simulink model "nms_model"  (R2020a)
settings: Solver=ode15s  StartTime=0.0  StopTime=2.6  MaxStep=.01  RelTol=1e-4  AbsTol=1e-6  EnableMultiTasking=on
values from neighbouring files (symbols this model uses):
  dt_visual = -1    [NMScontrol.m]    (also in runmodel.m = 0.001)
  g = params.g    [NMPCcostFunction.m]    (also in dynamicsNMPC.m = 9.81)
  m = parametersOpt(1)    [CGBgreybox.m]    (also in NMPCcostFunction.m = params.m)
undefined symbols (not defined in the file or in its folder): hatLeftHipToCenterDistWidth, initialTargetAngle, LongDelay, LongLoopDelay, LPreStimBFSHinit, LPreStimGASinit, LPreStimGLUinit, LPreStimHABinit, LPreStimHADinit, LPreStimHAMinit, LPreStimHFLinit, LPreStimRFinit, LPreStimSOLinit, LPreStimTAinit, LPreStimVASinit, LTargetAngleInit, LTargetAngleRInit, MidDelay, RPreStimBFSHinit, RPreStimGASinit, RPreStimGLUinit, RPreStimHABinit, RPreStimHADinit, RPreStimHAMinit, RPreStimHFLinit, RPreStimRFinit, RPreStimSOLinit, RPreStimTAinit, RPreStimVASinit, RTargetAngleInit, RTargetAngleRInit, ShortDelay, termination_height, thetaHATref, X, Y, Z
libraries: NeuroMuscularLibrary x107, nesl_utility x25, sm_lib x16, simulink x3
(part 1 of 3)
settings Model: SimulationMode=rapid-accelerator  ParamWorkspaceSource=ReferencedWorkspace  ExtModeTrigDuration=100  TunableVars=GainGAS,GainGLU,GainHAM,GainKneeOverExt,GainSOL,GainSOLTA,GainTA,GainVAS,Kglu,PosGainGG,SpeedGainGG,groundTheta,groundX,groundZ,hipDGain,hipPGain,kneeExtendGain,kneeFlexGain,kneeHoldGain1,kneeHoldGain2,kneeStopGain,legAngleFilter,legLengthClr,simbiconGainD,simbiconGainV,simbiconLegAngle0  TunableVarsStorageClass=Auto,Auto,Auto,Auto,Auto,Auto,Auto,Auto,Auto,Auto,Auto,Auto,Auto,Auto,Auto,Auto,Auto,Auto,Auto,Auto,Auto,Auto,Auto,Auto,Auto,Auto  TunableVarsTypeQualifier=,,,,,,,,,,,,,,,,,,,,,,,,,  Creator=nitisht  LastModifiedBy=Jesper
settings SolverCC: AutoScaleAbsTol=off  ZeroCrossAlgorithm=Adaptive
settings DataIOCC: LimitDataPoints=on  SaveFinalState=on  SaveFormat=StructureWithTime  SaveOutput=off  SaveState=on  ReturnWorkspaceOutputs=off  StateSaveName=tmp_raccel_xout  SignalLoggingName=tmp_raccel_logsout
settings OptimizationCC: DefaultParameterBehavior=Inlined  EfficientMapNaN2IntZero=off  LifeSpan=inf  SimCompilerOptimization=on
settings DebuggingCC: SaveWithDisabledLinksMsg=none  UnderspecifiedInitializationDetection=Classic  MergeDetectMultiDrivingBlocksExec=none  IgnoredZcDiagnostic=none  SolverPrmCheckMsg=warning  StateNameClashWarn=warning  SFUnexpectedBacktrackingDiag=warning  SFNoUnconditionalDefaultTransitionDiag=warning  SFExecutionAtInitializationDiag=none  ArithmeticOperatorsInVariantConditions=warning
settings HardwareCC: ProdBitPerPointer=32  ProdBitPerSizeT=32  ProdBitPerPtrDiffT=32  ProdLargestAtomicFloat=None  ProdIntDivRoundTo=Undefined  ProdEndianess=Unspecified  ProdWordSize=32  ProdHWDeviceType=Generic->Unspecified (assume 32-bit Generic)  TargetBitPerPointer=64  TargetBitPerSizeT=64  TargetBitPerPtrDiffT=64  TargetLongLongMode=on  TargetIntDivRoundTo=Zero  TargetEndianess=LittleEndian  TargetWordSize=64  TargetHWDeviceType=MATLAB Host  ProdEqTarget=off
settings ModelReferenceCC: PropagateSignalLabelsOutOfModel=off
settings SFSimCC: SFSimEcho=off  SimUseLocalCustomCode=off  CustomCodeUndefinedFunction=UseInterfaceOnly
settings RTWCC: SystemTargetFile=raccel.tlc  TemplateMakefile=raccel_default_tmf  RTWUseLocalCustomCode=off  RTWUseSimCustomCode=on
settings CodeAppCC: GenerateComments=off  MaxIdLength=128  MangleLength=10  SimulinkBlockComments=off
settings RaccelTargetCC: MultiInstanceERTCode=off  ENABLE_SLEXEC_SSBRIDGE=0  RTWCAPIParams=off  RTWCAPIRootIO=off
settings ConfigComp: CovMetricSettings=dw  CovHtmlReporting=on  CovSaveCumulativeToWorkspaceVar=on  CovSaveSingleToWorkspaceVar=on  CovExternalEMLEnable=off  CovSFcnEnable=off
settings SimscapeCC: SimscapeNormalizeSystem=off
settings ConfigurationSet: Description=SimMechanics 2G

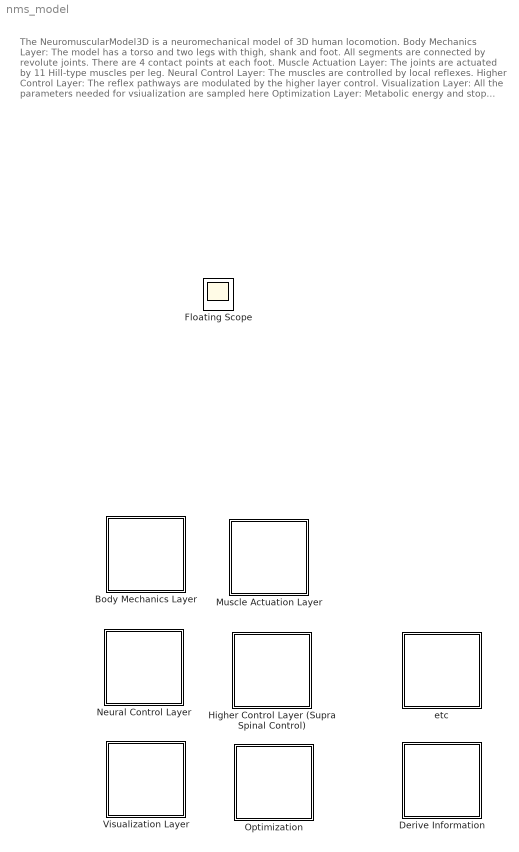
== system nms_model ==
  note: The NeuromuscularModel3D is a neuromechanical model of 3D human locomotion.
      |
      | Body Mechanics Layer:
      | The model has a torso and two legs with thigh, shank and foot.
      | All segments are connected by revolute joints.
      | There are 4 contact points at each foot.
      |
      | Muscle Actuation Layer:
      | The joints are actuated by 11 Hill-type muscles per leg.
      |
      | Neural Control Layer:
      | The muscles are controlled by local reflexes.
      |
      | Higher Control Layer:
      | The reflex pathways are modulated by the higher layer control.
      |
      | Visualization Layer:
      | All the parameters needed for vsiualization are sampled here
      |
      | Optimization Layer:
      | Metabolic energy and stop torques are calculated here.
      |
      | Derive Information Layer:
      | Contains gait phase detector, self collision detector, and step information calculator.
      |
      | Etc Layer:
      | Contains some stop conditions for when to stop simulation.
  Body Mechanics Layer : Subsystem
  Derive Information : Subsystem
  Higher Control Layer (Supra Spinal Control) : Subsystem
  Muscle Actuation Layer : Subsystem
  Neural Control Layer : Subsystem
  Optimization : Subsystem
  Visualization Layer : Subsystem
  etc : Subsystem
  Floating Scope : Scope

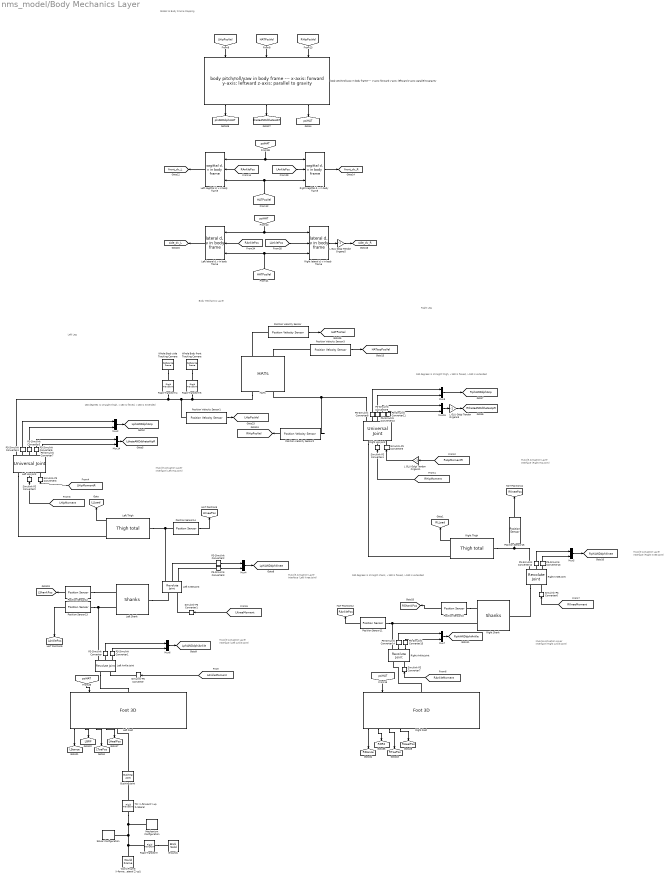
== system nms_model/Body Mechanics Layer ==
  note: 180 degrees is straight thigh, <180 is flexed, >180 is extended
  note: Body Mechanics Layer
  note: Left Leg
  note: Right Leg
  note: Muscle Actuation
      | Layer Interface
      | (Left Hip Joint)
  note: Muscle Actuation
      | Layer Interface
      | (Left Knee Joint)
  note: Muscle Actuation
      | Layer Interface
      | (Left Ankle Joint)
  note: Muscle Actuation
      | Layer Interface
      | (Right Ankle Joint)
  note: Muscle Actuation
      | Layer Interface
      | (Right Knee Joint)
  note: Muscle Actuation
      | Layer Interface
      | (Right Hip Joint)
  note: Global to Body Frame Mapping
  note: 180 degrees is straight thigh, <180 is flexed, >180 is extended
  note: 180 degrees is straight shank, <180 is flexed, >180 is extended
  Bushing Joint : sm_lib/Joints/Bushing Joint  JointMode=Normal  SenseConstraintForce=off  SenseConstraintForceX=off  SenseConstraintForceY=off  SenseConstraintForceZ=off  SenseConstraintTorque=off  SenseConstraintTorqueX=off  SenseConstraintTorqueY=off  SenseConstraintTorqueZ=off  SenseTotalForce=off  SenseTotalForceX=off  SenseTotalForceY=off  SenseTotalForceZ=off  SenseTotalTorque=off  SenseTotalTorqueX=off  SenseTotalTorqueY=off  SenseTotalTorqueZ=off  CompositeWrenchDir=FollowerOnBase  CompositeWrenchFrame=BaseFrame  PxEquilibriumPosition=0  PxEquilibriumPositionUnits=m  PxSpringStiffness=0  PxSpringStiffnessUnits=N/m  PxDampingCoefficient=0  PxDampingCoefficientUnits=N/(m/s)  PxTorqueActuationMode=NoTorque  PxMotionActuationMode=ComputedMotion  PxSensePosition=off  PxSenseVelocity=off  PxSenseAcceleration=off  PxSenseTorqueForce=off  PxSenseLowerLimitTorqueForce=off  PxSenseUpperLimitTorqueForce=off  PxLowerLimitSpecify=off  PxLowerLimitBound=-1  PxLowerLimitBoundUnits=m  PxLowerLimitStiffness=1e6  PxLowerLimitStiffnessUnits=N/m  PxLowerLimitDamping=1e3  PxLowerLimitDampingUnits=N/(m/s)  PxLowerLimitTransitionRegionWidth=1e-4  PxLowerLimitTransitionRegionWidthUnits=m  PxUpperLimitSpecify=off  PxUpperLimitBound=1  PxUpperLimitBoundUnits=m  PxUpperLimitStiffness=1e6  PxUpperLimitStiffnessUnits=N/m  PxUpperLimitDamping=1e3  PxUpperLimitDampingUnits=N/(m/s)  PxUpperLimitTransitionRegionWidth=1e-4  PxUpperLimitTransitionRegionWidthUnits=m  PxPositionTargetSpecify=on  PxPositionTargetPriority=High  PxPositionTargetValue=xInit  PxPositionTargetValueUnits=m  PxVelocityTargetSpecify=on  PxVelocityTargetPriority=High  PxVelocityTargetValue=vxInit  PxVelocityTargetValueUnits=m/s  PyEquilibriumPosition=0  PyEquilibriumPositionUnits=m  PySpringStiffness=0  PySpringStiffnessUnits=N/m  PyDampingCoefficient=0  PyDampingCoefficientUnits=N/(m/s)  PyTorqueActuationMode=NoTorque  PyMotionActuationMode=ComputedMotion  PySensePosition=off  PySenseVelocity=off  PySenseAcceleration=off  PySenseTorqueForce=off  PySenseLowerLimitTorqueForce=off  PySenseUpperLimitTorqueForce=off  PyLowerLimitSpecify=off  PyLowerLimitBound=-1  PyLowerLimitBoundUnits=m  PyLowerLimitStiffness=1e6  PyLowerLimitStiffnessUnits=N/m  PyLowerLimitDamping=1e3  PyLowerLimitDampingUnits=N/(m/s)  PyLowerLimitTransitionRegionWidth=1e-4  PyLowerLimitTransitionRegionWidthUnits=m  PyUpperLimitSpecify=off  PyUpperLimitBound=1  PyUpperLimitBoundUnits=m  PyUpperLimitStiffness=1e6  PyUpperLimitStiffnessUnits=N/m  PyUpperLimitDamping=1e3  PyUpperLimitDampingUnits=N/(m/s)  PyUpperLimitTransitionRegionWidth=1e-4  PyUpperLimitTransitionRegionWidthUnits=m  PyPositionTargetSpecify=on  PyPositionTargetPriority=High  PyPositionTargetValue=zInit  PyPositionTargetValueUnits=m  PyVelocityTargetSpecify=on  PyVelocityTargetPriority=High  PyVelocityTargetValue=vzInit  PyVelocityTargetValueUnits=m/s  PzEquilibriumPosition=0  PzEquilibriumPositionUnits=m  PzSpringStiffness=0  PzSpringStiffnessUnits=N/m  PzDampingCoefficient=0  PzDampingCoefficientUnits=N/(m/s)  PzTorqueActuationMode=NoTorque  PzMotionActuationMode=ComputedMotion  PzSensePosition=off  PzSenseVelocity=off  PzSenseAcceleration=off  PzSenseTorqueForce=off  PzSenseLowerLimitTorqueForce=off  PzSenseUpperLimitTorqueForce=off  PzLowerLimitSpecify=off  PzLowerLimitBound=-1  PzLowerLimitBoundUnits=m  PzLowerLimitStiffness=1e6  PzLowerLimitStiffnessUnits=N/m  PzLowerLimitDamping=1e3  PzLowerLimitDampingUnits=N/(m/s)  PzLowerLimitTransitionRegionWidth=1e-4  PzLowerLimitTransitionRegionWidthUnits=m  PzUpperLimitSpecify=off  PzUpperLimitBound=1  PzUpperLimitBoundUnits=m  PzUpperLimitStiffness=1e6  PzUpperLimitStiffnessUnits=N/m  PzUpperLimitDamping=1e3  PzUpperLimitDampingUnits=N/(m/s)  PzUpperLimitTransitionRegionWidth=1e-4  PzUpperLimitTransitionRegionWidthUnits=m  PzPositionTargetSpecify=on  PzPositionTargetPriority=High  PzPositionTargetValue=yInit  PzPositionTargetValueUnits=m  PzVelocityTargetSpecify=on  PzVelocityTargetPriority=High  PzVelocityTargetValue=vyInit  PzVelocityTargetValueUnits=m/s  RxEquilibriumPosition=0  RxEquilibriumPositionUnits=deg  RxSpringStiffness=0  RxSpringStiffnessUnits=N*m/deg  RxDampingCoefficient=0  RxDampingCoefficientUnits=N*m/(deg/s)  RxTorqueActuationMode=NoTorque  RxMotionActuationMode=ComputedMotion  RxSensePosition=off  RxSenseVelocity=off  RxSenseAcceleration=off  RxSenseTorqueForce=off  RxSenseLowerLimitTorqueForce=off  RxSenseUpperLimitTorqueForce=off  RxLowerLimitSpecify=off  RxLowerLimitBound=-90  RxLowerLimitBoundUnits=deg  RxLowerLimitStiffness=1e4  RxLowerLimitStiffnessUnits=N*m/deg  RxLowerLimitDamping=10  RxLowerLimitDampingUnits=N*m/(deg/s)  RxLowerLimitTransitionRegionWidth=0.1  RxLowerLimitTransitionRegionWidthUnits=deg  RxUpperLimitSpecify=off  RxUpperLimitBound=90  RxUpperLimitBoundUnits=deg  RxUpperLimitStiffness=1e4  RxUpperLimitStiffnessUnits=N*m/deg  RxUpperLimitDamping=10  RxUpperLimitDampingUnits=N*m/(deg/s)  RxUpperLimitTransitionRegionWidth=0.1  RxUpperLimitTransitionRegionWidthUnits=deg  RxPositionTargetSpecify=on  RxPositionTargetPriority=High  RxPositionTargetValue=rollInit  RxPositionTargetValueUnits=rad  RxVelocityTargetSpecify=on  RxVelocityTargetPriority=High  RxVelocityTargetValue=0  RxVelocityTargetValueUnits=rad/s  RyEquilibriumPosition=0  RyEquilibriumPositionUnits=deg  RySpringStiffness=0  RySpringStiffnessUnits=N*m/deg  RyDampingCoefficient=0  RyDampingCoefficientUnits=N*m/(deg/s)  RyTorqueActuationMode=NoTorque  RyMotionActuationMode=ComputedMotion  RySensePosition=off  RySenseVelocity=off  RySenseAcceleration=off  RySenseTorqueForce=off  RySenseLowerLimitTorqueForce=off  RySenseUpperLimitTorqueForce=off  RyLowerLimitSpecify=off  RyLowerLimitBound=-90  RyLowerLimitBoundUnits=deg  RyLowerLimitStiffness=1e4  RyLowerLimitStiffnessUnits=N*m/deg  RyLowerLimitDamping=10  RyLowerLimitDampingUnits=N*m/(deg/s)  RyLowerLimitTransitionRegionWidth=0.1  RyLowerLimitTransitionRegionWidthUnits=deg  RyUpperLimitSpecify=off  RyUpperLimitBound=90  RyUpperLimitBoundUnits=deg  RyUpperLimitStiffness=1e4  RyUpperLimitStiffnessUnits=N*m/deg  RyUpperLimitDamping=10  RyUpperLimitDampingUnits=N*m/(deg/s)  RyUpperLimitTransitionRegionWidth=0.1  RyUpperLimitTransitionRegionWidthUnits=deg  RyPositionTargetSpecify=on  RyPositionTargetPriority=High  RyPositionTargetValue=yawInit  RyPositionTargetValueUnits=rad  RyVelocityTargetSpecify=on  RyVelocityTargetPriority=High  RyVelocityTargetValue=0  RyVelocityTargetValueUnits=rad/s  RzEquilibriumPosition=0  RzEquilibriumPositionUnits=deg  RzSpringStiffness=0  RzSpringStiffnessUnits=N*m/deg  RzDampingCoefficient=0  RzDampingCoefficientUnits=N*m/(deg/s)  RzTorqueActuationMode=NoTorque  RzMotionActuationMode=ComputedMotion  RzSensePosition=off  RzSenseVelocity=off  RzSenseAcceleration=off  RzSenseTorqueForce=off  RzSenseLowerLimitTorqueForce=off  RzSenseUpperLimitTorqueForce=off  RzLowerLimitSpecify=off  RzLowerLimitBound=-90  RzLowerLimitBoundUnits=deg  RzLowerLimitStiffness=1e4  RzLowerLimitStiffnessUnits=N*m/deg  RzLowerLimitDamping=10  RzLowerLimitDampingUnits=N*m/(deg/s)  RzLowerLimitTransitionRegionWidth=0.1  RzLowerLimitTransitionRegionWidthUnits=deg  RzUpperLimitSpecify=off  RzUpperLimitBound=90  RzUpperLimitBoundUnits=deg  RzUpperLimitStiffness=1e4  RzUpperLimitStiffnessUnits=N*m/deg  RzUpperLimitDamping=10  RzUpperLimitDampingUnits=N*m/(deg/s)  RzUpperLimitTransitionRegionWidth=0.1  RzUpperLimitTransitionRegionWidthUnits=deg  RzPositionTargetSpecify=off  RzPositionTargetPriority=High  RzPositionTargetValue=0  RzPositionTargetValueUnits=deg  RzVelocityTargetSpecify=off  RzVelocityTargetPriority=High  RzVelocityTargetValue=0  RzVelocityTargetValueUnits=deg/s
  Ground1 : sm_lib/Body Elements/Brick Solid  GraphicAmbientColor=[0.15 0.15 0.15 1.0]  BasedOnType=Density  BrickDimensions=[3 1 .01]  BrickDimensionUnits=m  CenterOfMass=[0 0 0]  CenterOfMassUnits=m  GraphicDiffuseColor=[0.4 0.2 0.0]  Density=1000  DensityUnits=kg/(m^3)  DoExposeReferenceFrame=on  GraphicEmissiveColor=[0.0 0.0 0.0 1.0]  ExportEntireGeometry=off  SerializedFrames=<Frames/>  MarkerShape=Sphere  MarkerSize=10  GraphicType=FromGeometry  InertiaType=Custom  Mass=0  MassUnits=kg  MomentsOfInertia=[0 0 0]  MomentsOfInertiaUnits=kg*m^2  GraphicOpacity=1.0  ProductsOfInertia=[0 0 0]  ProductsOfInertiaUnits=kg*m^2  GraphicShininess=75  GraphicSpecularColor=[0.5 0.5 0.5 1.0]  GraphicVisPropType=SimpleVisualProperties
  HATs : NeuroMuscularLibrary/HATs  SystemSampleTime=-1  Latency=0  AutoFrameSizeCalculation=off
  L GLU Golgi Tendon Organs1 : Gain  Gain=-1
  L GLU Golgi Tendon Organs3 : Gain  Gain=-1
  L GLU Golgi Tendon Organs5 : Gain  Gain=-1
  Left Knee Joint : sm_lib/Joints/Revolute Joint  JointMode=Normal  SenseConstraintForce=off  SenseConstraintForceX=off  SenseConstraintForceY=off  SenseConstraintForceZ=off  SenseConstraintTorque=off  SenseConstraintTorqueX=off  SenseConstraintTorqueY=off  SenseConstraintTorqueZ=off  SenseTotalForce=off  SenseTotalForceX=off  SenseTotalForceY=off  SenseTotalForceZ=off  SenseTotalTorque=off  SenseTotalTorqueX=off  SenseTotalTorqueY=off  SenseTotalTorqueZ=off  CompositeWrenchDir=FollowerOnBase  CompositeWrenchFrame=BaseFrame  EquilibriumPosition=0  EquilibriumPositionUnits=deg  SpringStiffness=0  SpringStiffnessUnits=N*m/deg  DampingCoefficient=0  DampingCoefficientUnits=N*m/(deg/s)  TorqueActuationMode=InputTorque  MotionActuationMode=ComputedMotion  SensePosition=on  SenseVelocity=on  SenseAcceleration=off  SenseTorqueForce=off  SenseLowerLimitTorqueForce=off  SenseUpperLimitTorqueForce=off  LowerLimitSpecify=off  LowerLimitBound=-90  LowerLimitBoundUnits=deg  LowerLimitStiffness=1e4  LowerLimitStiffnessUnits=N*m/deg  LowerLimitDamping=10  LowerLimitDampingUnits=N*m/(deg/s)  LowerLimitTransitionRegionWidth=0.1  LowerLimitTransitionRegionWidthUnits=deg  UpperLimitSpecify=off  UpperLimitBound=90  UpperLimitBoundUnits=deg  UpperLimitStiffness=1e4  UpperLimitStiffnessUnits=N*m/deg  UpperLimitDamping=10  UpperLimitDampingUnits=N*m/(deg/s)  UpperLimitTransitionRegionWidth=0.1  UpperLimitTransitionRegionWidthUnits=deg  PositionTargetSpecify=on  PositionTargetPriority=High  PositionTargetValue=LphiKnee0  PositionTargetValueUnits=rad  VelocityTargetSpecify=on  VelocityTargetPriority=High  VelocityTargetValue=0  VelocityTargetValueUnits=rad/s
  Left Ankle joint : sm_lib/Joints/Revolute Joint  JointMode=Normal  SenseConstraintForce=off  SenseConstraintForceX=off  SenseConstraintForceY=off  SenseConstraintForceZ=off  SenseConstraintTorque=off  SenseConstraintTorqueX=off  SenseConstraintTorqueY=off  SenseConstraintTorqueZ=off  SenseTotalForce=off  SenseTotalForceX=off  SenseTotalForceY=off  SenseTotalForceZ=off  SenseTotalTorque=off  SenseTotalTorqueX=off  SenseTotalTorqueY=off  SenseTotalTorqueZ=off  CompositeWrenchDir=FollowerOnBase  CompositeWrenchFrame=BaseFrame  EquilibriumPosition=0  EquilibriumPositionUnits=deg  SpringStiffness=0  SpringStiffnessUnits=N*m/deg  DampingCoefficient=0  DampingCoefficientUnits=N*m/(deg/s)  TorqueActuationMode=InputTorque  MotionActuationMode=ComputedMotion  SensePosition=on  SenseVelocity=on  SenseAcceleration=off  SenseTorqueForce=off  SenseLowerLimitTorqueForce=off  SenseUpperLimitTorqueForce=off  LowerLimitSpecify=off  LowerLimitBound=-90  LowerLimitBoundUnits=deg  LowerLimitStiffness=1e4  LowerLimitStiffnessUnits=N*m/deg  LowerLimitDamping=10  LowerLimitDampingUnits=N*m/(deg/s)  LowerLimitTransitionRegionWidth=0.1  LowerLimitTransitionRegionWidthUnits=deg  UpperLimitSpecify=off  UpperLimitBound=90  UpperLimitBoundUnits=deg  UpperLimitStiffness=1e4  UpperLimitStiffnessUnits=N*m/deg  UpperLimitDamping=10  UpperLimitDampingUnits=N*m/(deg/s)  UpperLimitTransitionRegionWidth=0.1  UpperLimitTransitionRegionWidthUnits=deg  PositionTargetSpecify=on  PositionTargetPriority=High  PositionTargetValue=LphiAnkle0  PositionTargetValueUnits=rad  VelocityTargetSpecify=on  VelocityTargetPriority=High  VelocityTargetValue=0  VelocityTargetValueUnits=rad/s
  Left Foot : NeuroMuscularLibrary/Foot 3D  footMass=footMass  footInertia=footInertia  footSide=Left foot
  Left Hip Joint : sm_lib/Joints/Universal Joint  JointMode=Normal  SenseConstraintForce=off  SenseConstraintForceX=off  SenseConstraintForceY=off  SenseConstraintForceZ=off  SenseConstraintTorque=off  SenseConstraintTorqueX=off  SenseConstraintTorqueY=off  SenseConstraintTorqueZ=off  SenseTotalForce=off  SenseTotalForceX=off  SenseTotalForceY=off  SenseTotalForceZ=off  SenseTotalTorque=off  SenseTotalTorqueX=off  SenseTotalTorqueY=off  SenseTotalTorqueZ=off  CompositeWrenchDir=FollowerOnBase  CompositeWrenchFrame=BaseFrame  RxEquilibriumPosition=0  RxEquilibriumPositionUnits=deg  RxSpringStiffness=0  RxSpringStiffnessUnits=N*m/deg  RxDampingCoefficient=0  RxDampingCoefficientUnits=N*m/(deg/s)  RxTorqueActuationMode=InputTorque  RxMotionActuationMode=ComputedMotion  RxSensePosition=on  RxSenseVelocity=on  RxSenseAcceleration=off  RxSenseTorqueForce=off  RxSenseLowerLimitTorqueForce=off  RxSenseUpperLimitTorqueForce=off  RxLowerLimitSpecify=off  RxLowerLimitBound=-90  RxLowerLimitBoundUnits=deg  RxLowerLimitStiffness=1e4  RxLowerLimitStiffnessUnits=N*m/deg  RxLowerLimitDamping=10  RxLowerLimitDampingUnits=N*m/(deg/s)  RxLowerLimitTransitionRegionWidth=0.1  RxLowerLimitTransitionRegionWidthUnits=deg  RxUpperLimitSpecify=off  RxUpperLimitBound=90  RxUpperLimitBoundUnits=deg  RxUpperLimitStiffness=1e4  RxUpperLimitStiffnessUnits=N*m/deg  RxUpperLimitDamping=10  RxUpperLimitDampingUnits=N*m/(deg/s)  RxUpperLimitTransitionRegionWidth=0.1  RxUpperLimitTransitionRegionWidthUnits=deg  RxPositionTargetSpecify=on  RxPositionTargetPriority=High  RxPositionTargetValue=LphiHip0  RxPositionTargetValueUnits=rad  RxVelocityTargetSpecify=on  RxVelocityTargetPriority=High  RxVelocityTargetValue=0  RxVelocityTargetValueUnits=rad/s  RyEquilibriumPosition=0  RyEquilibriumPositionUnits=deg  RySpringStiffness=0  RySpringStiffnessUnits=N*m/deg  RyDampingCoefficient=0  RyDampingCoefficientUnits=N*m/(deg/s)  RyTorqueActuationMode=InputTorque  RyMotionActuationMode=ComputedMotion  RySensePosition=on  RySenseVelocity=on  RySenseAcceleration=off  RySenseTorqueForce=off  RySenseLowerLimitTorqueForce=off  RySenseUpperLimitTorqueForce=off  RyLowerLimitSpecify=off  RyLowerLimitBound=-90  RyLowerLimitBoundUnits=deg  RyLowerLimitStiffness=1e4  RyLowerLimitStiffnessUnits=N*m/deg  RyLowerLimitDamping=10  RyLowerLimitDampingUnits=N*m/(deg/s)  RyLowerLimitTransitionRegionWidth=0.1  RyLowerLimitTransitionRegionWidthUnits=deg  RyUpperLimitSpecify=off  RyUpperLimitBound=90  RyUpperLimitBoundUnits=deg  RyUpperLimitStiffness=1e4  RyUpperLimitStiffnessUnits=N*m/deg  RyUpperLimitDamping=10  RyUpperLimitDampingUnits=N*m/(deg/s)  RyUpperLimitTransitionRegionWidth=0.1  RyUpperLimitTransitionRegionWidthUnits=deg  RyPositionTargetSpecify=on  RyPositionTargetPriority=High  RyPositionTargetValue=LphiHipR0  RyPositionTargetValueUnits=rad  RyVelocityTargetSpecify=on  RyVelocityTargetPriority=High  RyVelocityTargetValue=0  RyVelocityTargetValueUnits=rad/s
  Left Shank : NeuroMuscularLibrary/Shanks  SystemSampleTime=-1  Latency=0  AutoFrameSizeCalculation=off
  Left Thigh : NeuroMuscularLibrary/Thigh total  SystemSampleTime=-1  Latency=0  AutoFrameSizeCalculation=off
  "Left lateral d, v in body frame" : NeuroMuscularLibrary/lateral d, v in body frame  SystemSampleTime=-1  Latency=0  AutoFrameSizeCalculation=off
  "Left sagittal d, v in body frame" : NeuroMuscularLibrary/sagittal d, v in body frame  SystemSampleTime=-1  Latency=0  AutoFrameSizeCalculation=off
  Mechanism Configuration : sm_lib/Utilities/Mechanism Configuration  UniformGravity=Constant  GravityVector=[0 0 -g]  GravityUnits=m/s^2  LinearizationDelta=0.001
  Mux{2..7,14..15} (8 alike) : Mux  Inputs=2
  PS-Simulink Converter{,2,4,6,8,10,12,14} (8 alike) : nesl_utility/PS-Simulink Converter  PhysicalDomain=network_engine_domain  SubClassName=ps_output  LeftPortType=input  RightPortType=output  PseudoPeriodic=off  Frequencies=[]  Unit=rad  AffineConversion=off
  PS-Simulink Converter{1,3,5,7,9,11,13,15} (8 alike) : nesl_utility/PS-Simulink Converter  PhysicalDomain=network_engine_domain  SubClassName=ps_output  LeftPortType=input  RightPortType=output  PseudoPeriodic=off  Frequencies=[]  Unit=rad/s  AffineConversion=off
  Position Sensor{10..15} (6 alike) : NeuroMuscularLibrary/Position Sensor  SystemSampleTime=-1  Latency=0  AutoFrameSizeCalculation=off
  Position Velocity Sensor{,1..3} (4 alike) : NeuroMuscularLibrary/Position Velocity Sensor  SystemSampleTime=-1  Latency=0  AutoFrameSizeCalculation=off
  Right Ankle Joint : sm_lib/Joints/Revolute Joint  JointMode=Normal  SenseConstraintForce=off  SenseConstraintForceX=off  SenseConstraintForceY=off  SenseConstraintForceZ=off  SenseConstraintTorque=off  SenseConstraintTorqueX=off  SenseConstraintTorqueY=off  SenseConstraintTorqueZ=off  SenseTotalForce=off  SenseTotalForceX=off  SenseTotalForceY=off  SenseTotalForceZ=off  SenseTotalTorque=off  SenseTotalTorqueX=off  SenseTotalTorqueY=off  SenseTotalTorqueZ=off  CompositeWrenchDir=FollowerOnBase  CompositeWrenchFrame=BaseFrame  EquilibriumPosition=0  EquilibriumPositionUnits=deg  SpringStiffness=0  SpringStiffnessUnits=N*m/deg  DampingCoefficient=0  DampingCoefficientUnits=N*m/(deg/s)  TorqueActuationMode=InputTorque  MotionActuationMode=ComputedMotion  SensePosition=on  SenseVelocity=on  SenseAcceleration=off  SenseTorqueForce=off  SenseLowerLimitTorqueForce=off  SenseUpperLimitTorqueForce=off  LowerLimitSpecify=off  LowerLimitBound=-90  LowerLimitBoundUnits=deg  LowerLimitStiffness=1e4  LowerLimitStiffnessUnits=N*m/deg  LowerLimitDamping=10  LowerLimitDampingUnits=N*m/(deg/s)  LowerLimitTransitionRegionWidth=0.1  LowerLimitTransitionRegionWidthUnits=deg  UpperLimitSpecify=off  UpperLimitBound=90  UpperLimitBoundUnits=deg  UpperLimitStiffness=1e4  UpperLimitStiffnessUnits=N*m/deg  UpperLimitDamping=10  UpperLimitDampingUnits=N*m/(deg/s)  UpperLimitTransitionRegionWidth=0.1  UpperLimitTransitionRegionWidthUnits=deg  PositionTargetSpecify=on  PositionTargetPriority=High  PositionTargetValue=RphiAnkle0  PositionTargetValueUnits=rad  VelocityTargetSpecify=on  VelocityTargetPriority=High  VelocityTargetValue=0  VelocityTargetValueUnits=rad/s
  Right Foot : NeuroMuscularLibrary/Foot 3D  footMass=footMass  footInertia=footInertia  footSide=Right foot
  Right Hip joint : sm_lib/Joints/Universal Joint  JointMode=Normal  SenseConstraintForce=off  SenseConstraintForceX=off  SenseConstraintForceY=off  SenseConstraintForceZ=off  SenseConstraintTorque=off  SenseConstraintTorqueX=off  SenseConstraintTorqueY=off  SenseConstraintTorqueZ=off  SenseTotalForce=off  SenseTotalForceX=off  SenseTotalForceY=off  SenseTotalForceZ=off  SenseTotalTorque=off  SenseTotalTorqueX=off  SenseTotalTorqueY=off  SenseTotalTorqueZ=off  CompositeWrenchDir=FollowerOnBase  CompositeWrenchFrame=BaseFrame  RxEquilibriumPosition=0  RxEquilibriumPositionUnits=deg  RxSpringStiffness=0  RxSpringStiffnessUnits=N*m/deg  RxDampingCoefficient=0  RxDampingCoefficientUnits=N*m/(deg/s)  RxTorqueActuationMode=InputTorque  RxMotionActuationMode=ComputedMotion  RxSensePosition=on  RxSenseVelocity=on  RxSenseAcceleration=off  RxSenseTorqueForce=off  RxSenseLowerLimitTorqueForce=off  RxSenseUpperLimitTorqueForce=off  RxLowerLimitSpecify=off  RxLowerLimitBound=-90  RxLowerLimitBoundUnits=deg  RxLowerLimitStiffness=1e4  RxLowerLimitStiffnessUnits=N*m/deg  RxLowerLimitDamping=10  RxLowerLimitDampingUnits=N*m/(deg/s)  RxLowerLimitTransitionRegionWidth=0.1  RxLowerLimitTransitionRegionWidthUnits=deg  RxUpperLimitSpecify=off  RxUpperLimitBound=90  RxUpperLimitBoundUnits=deg  RxUpperLimitStiffness=1e4  RxUpperLimitStiffnessUnits=N*m/deg  RxUpperLimitDamping=10  RxUpperLimitDampingUnits=N*m/(deg/s)  RxUpperLimitTransitionRegionWidth=0.1  RxUpperLimitTransitionRegionWidthUnits=deg  RxPositionTargetSpecify=on  RxPositionTargetPriority=High  RxPositionTargetValue=RphiHip0  RxPositionTargetValueUnits=rad  RxVelocityTargetSpecify=on  RxVelocityTargetPriority=High  RxVelocityTargetValue=0  RxVelocityTargetValueUnits=rad/s  RyEquilibriumPosition=0  RyEquilibriumPositionUnits=deg  RySpringStiffness=0  RySpringStiffnessUnits=N*m/deg  RyDampingCoefficient=0  RyDampingCoefficientUnits=N*m/(deg/s)  RyTorqueActuationMode=InputTorque  RyMotionActuationMode=ComputedMotion  RySensePosition=on  RySenseVelocity=on  RySenseAcceleration=off  RySenseTorqueForce=off  RySenseLowerLimitTorqueForce=off  RySenseUpperLimitTorqueForce=off  RyLowerLimitSpecify=off  RyLowerLimitBound=-90  RyLowerLimitBoundUnits=deg  RyLowerLimitStiffness=1e4  RyLowerLimitStiffnessUnits=N*m/deg  RyLowerLimitDamping=10  RyLowerLimitDampingUnits=N*m/(deg/s)  RyLowerLimitTransitionRegionWidth=0.1  RyLowerLimitTransitionRegionWidthUnits=deg  RyUpperLimitSpecify=off  RyUpperLimitBound=90  RyUpperLimitBoundUnits=deg  RyUpperLimitStiffness=1e4  RyUpperLimitStiffnessUnits=N*m/deg  RyUpperLimitDamping=10  RyUpperLimitDampingUnits=N*m/(deg/s)  RyUpperLimitTransitionRegionWidth=0.1  RyUpperLimitTransitionRegionWidthUnits=deg  RyPositionTargetSpecify=on  RyPositionTargetPriority=High  RyPositionTargetValue=RphiHipR0  RyPositionTargetValueUnits=rad  RyVelocityTargetSpecify=on  RyVelocityTargetPriority=High  RyVelocityTargetValue=0  RyVelocityTargetValueUnits=rad/s
  Right Knee joint : sm_lib/Joints/Revolute Joint  JointMode=Normal  SenseConstraintForce=off  SenseConstraintForceX=off  SenseConstraintForceY=off  SenseConstraintForceZ=off  SenseConstraintTorque=off  SenseConstraintTorqueX=off  SenseConstraintTorqueY=off  SenseConstraintTorqueZ=off  SenseTotalForce=off  SenseTotalForceX=off  SenseTotalForceY=off  SenseTotalForceZ=off  SenseTotalTorque=off  SenseTotalTorqueX=off  SenseTotalTorqueY=off  SenseTotalTorqueZ=off  CompositeWrenchDir=FollowerOnBase  CompositeWrenchFrame=BaseFrame  EquilibriumPosition=0  EquilibriumPositionUnits=deg  SpringStiffness=0  SpringStiffnessUnits=N*m/deg  DampingCoefficient=0  DampingCoefficientUnits=N*m/(deg/s)  TorqueActuationMode=InputTorque  MotionActuationMode=ComputedMotion  SensePosition=on  SenseVelocity=on  SenseAcceleration=off  SenseTorqueForce=off  SenseLowerLimitTorqueForce=off  SenseUpperLimitTorqueForce=off  LowerLimitSpecify=off  LowerLimitBound=-90  LowerLimitBoundUnits=deg  LowerLimitStiffness=1e4  LowerLimitStiffnessUnits=N*m/deg  LowerLimitDamping=10  LowerLimitDampingUnits=N*m/(deg/s)  LowerLimitTransitionRegionWidth=0.1  LowerLimitTransitionRegionWidthUnits=deg  UpperLimitSpecify=off  UpperLimitBound=90  UpperLimitBoundUnits=deg  UpperLimitStiffness=1e4  UpperLimitStiffnessUnits=N*m/deg  UpperLimitDamping=10  UpperLimitDampingUnits=N*m/(deg/s)  UpperLimitTransitionRegionWidth=0.1  UpperLimitTransitionRegionWidthUnits=deg  PositionTargetSpecify=on  PositionTargetPriority=High  PositionTargetValue=RphiKnee0  PositionTargetValueUnits=rad  VelocityTargetSpecify=on  VelocityTargetPriority=High  VelocityTargetValue=0  VelocityTargetValueUnits=rad/s
  Right Shank : NeuroMuscularLibrary/Shanks  SystemSampleTime=-1  Latency=0  AutoFrameSizeCalculation=off
  Right Thigh : NeuroMuscularLibrary/Thigh total  SystemSampleTime=-1  Latency=0  AutoFrameSizeCalculation=off
  "Right lateral d, v in body frame" : NeuroMuscularLibrary/lateral d, v in body frame  SystemSampleTime=-1  Latency=0  AutoFrameSizeCalculation=off
  "Right sagittal d, v in body frame" : NeuroMuscularLibrary/sagittal d, v in body frame  SystemSampleTime=-1  Latency=0  AutoFrameSizeCalculation=off
  Rigid Transform4 : sm_lib/Frames and Transforms/Rigid Transform  TranslationMethod=Cartesian  TranslationStandardOffset=3  TranslationLengthUnit=m  TranslationStandardAxis=+Z  TranslationCartesianOffset=[ 2.5 0 0]  TranslationROffset=0  TranslationROffsetUnits=m  TranslationZOffset=0  TranslationZOffsetUnits=m  TranslationThetaOffset=0  TranslationThetaOffsetUnits=deg  RotationMethod=None  RotationAngleUnits=deg  RotationStandardAxis=+Z  RotationAngle=0.0  RotationArbitraryAxis=[0 0 1]  FollAlignAxisA=+X  BaseAlignAxisA=+Y  FollAlignAxisB=+Y  BaseAlignAxisB=+Z  RotationSequenceAxes=FollowerAxes  RotationSequence=XYX  RotationSequenceAngles=[0 0 0]  RotationSequenceAnglesUnits=deg  RotationMatrix=[1 0 0; 0 1 0; 0 0 1]
  Rigid Transform5 : sm_lib/Frames and Transforms/Rigid Transform  TranslationMethod=Cartesian  TranslationStandardOffset=3  TranslationLengthUnit=m  TranslationStandardAxis=+Z  TranslationCartesianOffset=[0.2 -3 -1.3]  TranslationROffset=0  TranslationROffsetUnits=m  TranslationZOffset=0  TranslationZOffsetUnits=m  TranslationThetaOffset=0  TranslationThetaOffsetUnits=deg  RotationMethod=None  RotationAngleUnits=deg  RotationStandardAxis=+Z  RotationAngle=0.0  RotationArbitraryAxis=[0 0 1]  FollAlignAxisA=+X  BaseAlignAxisA=+Y  FollAlignAxisB=+Y  BaseAlignAxisB=+Z  RotationSequenceAxes=FollowerAxes  RotationSequence=XYX  RotationSequenceAngles=[0 0 0]  RotationSequenceAnglesUnits=deg  RotationMatrix=[1 0 0; 0 1 0; 0 0 1]
  Rigid Transform : sm_lib/Frames and Transforms/Rigid Transform  TranslationMethod=Cartesian  TranslationStandardOffset=1  TranslationLengthUnit=m  TranslationStandardAxis=+X  TranslationCartesianOffset="[1  0 0]"  TranslationROffset=0  TranslationROffsetUnits=m  TranslationZOffset=0  TranslationZOffsetUnits=m  TranslationThetaOffset=0  TranslationThetaOffsetUnits=deg  RotationMethod=None  RotationAngleUnits=deg  RotationStandardAxis=+Z  RotationAngle=0  RotationArbitraryAxis=[0 0 1]  FollAlignAxisA=+X  BaseAlignAxisA=+Y  FollAlignAxisB=+Y  BaseAlignAxisB=+Z  RotationSequenceAxes=FollowerAxes  RotationSequence=XYX  RotationSequenceAngles=[0 0 0]  RotationSequenceAnglesUnits=deg  RotationMatrix=[1 0 0; 0 1 0; 0 0 1]
  Simulink-PS Converter{,1..6} (7 alike) : nesl_utility/Simulink-PS Converter  PhysicalDomain=network_engine_domain  SubClassName=ps_input  LeftPortType=input  RightPortType=output  PseudoPeriodic=off  Frequencies=[]  NoiseDistribution=none  NoiseParameters=[]  Unit=N*m  AffineConversion=off  FilteringAndDerivatives=provide  SimscapeFilterOrder=1  InputFilterTimeConstant=0.001  UdotUserProvided=0
  Simulink-PS Converter7 : nesl_utility/Simulink-PS Converter  PhysicalDomain=network_engine_domain  SubClassName=ps_input  LeftPortType=input  RightPortType=output  PseudoPeriodic=off  Frequencies=[]  NoiseDistribution=none  NoiseParameters=[]  Unit=1  AffineConversion=off  FilteringAndDerivatives=provide  SimscapeFilterOrder=1  InputFilterTimeConstant=0.001  UdotUserProvided=0
  Solver Configuration : nesl_utility/Solver Configuration  PhysicalDomain=network_engine_domain  SubClassName=solver  LeftPortType=input  RightPortType=generic  Tones=[]  Harmonics=[]  SimulateNoise=off  Profile=off  UseLocalSampling=off  EnableSwitchedLinearOptims=on  FrequencyDomain=off  UseCCode=off  RelTol=0.001  AbsTol=1e-06  MinStep=1e-09  ToWorkspace=off  RevertToSquareIcSolve=off  NumHomotopyIterations=100  PhasorMode=off  PhasorModeNumHarmonics=1  DoDC=off  ResidualTolerance=1e-09  UseLocalSolver=off  LocalSolverChoice=NE_BACKWARD_EULER_ADVANCER  LocalSolverSampleTime=0.001  DoFixedCost=off  MaxNonlinIter=3  MaxModeIter=2  LinearAlgebra=Sparse  EquationFormulation=NE_TIME_EF  DelaysMemoryBudget=1024  AutomaticFiltering=on  FilteringTimeConstant=0.001  PartitionStorageMethod=AS_NEEDED  PartitionMemoryBudget=1024  PartitionMethod=FAST
  TO: X-forward Y-up Z-lateral : sm_lib/Frames and Transforms/Rigid Transform  TranslationMethod=StandardAxis  TranslationStandardOffset=hatLeftHipToCenterDistWidth/2  TranslationLengthUnit=m  TranslationStandardAxis=+Z  TranslationCartesianOffset=[0 0 0]  TranslationROffset=0  TranslationROffsetUnits=m  TranslationZOffset=0  TranslationZOffsetUnits=m  TranslationThetaOffset=0  TranslationThetaOffsetUnits=deg  RotationMethod=AlignedAxes  RotationAngleUnits=deg  RotationStandardAxis=+Z  RotationAngle=0  RotationArbitraryAxis=[0 0 1]  FollAlignAxisA=+Z  BaseAlignAxisA=+Y  FollAlignAxisB=+X  BaseAlignAxisB=+X  RotationSequenceAxes=FollowerAxes  RotationSequence=XYX  RotationSequenceAngles=[0 0 0]  RotationSequenceAnglesUnits=deg  RotationMatrix=[1 0 0; 0 1 0; 0 0 1]
  Whole Body front Tracking Camera : sm_lib/Frames and Transforms/Reference Frame
  Whole Body side Tracking Camera : sm_lib/Frames and Transforms/Reference Frame
  World Frame X-forward Y-lateral Z-up1 : sm_lib/Frames and Transforms/World Frame
  body pitch/roll/yaw in body frame --- x-axis: forward y-axis: leftward z-axis: parallel to gravity : NeuroMuscularLibrary/body pitch//roll//yaw in body frame --- x-axis: forward y-axis: leftward z-axis: parallel to gravity  SystemSampleTime=-1  Latency=0  AutoFrameSizeCalculation=off
  tag scope: HATPosVel=global, HATtopPosVel=global, LAnklePos=global, LGRF=global, LHeelPos=global, LHipPosVel=global, LKneePos=global, LLLoad=global, LShankPos=global, LStance=global, LToePos=global, LphiANDdphiAnkle=global, LphiANDdphiHip=global, LphiANDdphiKnee=global, LthetaANDdthetaHipR=global, RAnklePos=global, RGRF=global, RHeelPos=global, RHipPosVel=global, RKneePos=global, RLLoad=global, RShankPos=global, RStance=global, RToePos=global, RphiANDdphiAnkle=global, RphiANDdphiHip=global, RphiANDdphiKnee=global, RthetaANDdthetaHipR=global, front_dv_L=global, front_dv_R=global, phiANDdphiHAT=global, psiHAT=global, side_dv_L=global, side_dv_R=global, thetaANDdthetaHAT=global
  wires:
  PS-Simulink Converter2/1 -> Mux4/1
  PS-Simulink Converter3/1 -> Mux4/2
  Mux4/1 -> [LphiANDdphiKnee]
  PS-Simulink Converter/1 -> Mux6/1
  PS-Simulink Converter1/1 -> Mux6/2
  Mux6/1 -> [LphiANDdphiAnkle]
  Position Sensor13/1 -> [LAnklePos]
  [RAnkleMoment] -> Simulink-PS Converter7/1
  PS-Simulink Converter12/1 -> Mux5/1
  PS-Simulink Converter13/1 -> Mux5/2
  Mux5/1 -> [RphiANDdphiKnee]
  PS-Simulink Converter14/1 -> Mux7/1
  PS-Simulink Converter15/1 -> Mux7/2
  Mux7/1 -> [RphiANDdphiAnkle]
  Position Sensor15/1 -> [RKneePos]
  Position Sensor11/1 -> [RAnklePos]
  [LHipMoment] -> Simulink-PS Converter2/1
  PS-Simulink Converter4/1 -> Mux2/1
  PS-Simulink Converter5/1 -> Mux2/2
  Mux2/1 -> [LphiANDdphiHip]
  PS-Simulink Converter7/1 -> Mux14/2
  PS-Simulink Converter6/1 -> Mux14/1
  Mux14/1 -> [LthetaANDdthetaHipR]
  [LHipMomentR] -> Simulink-PS Converter3/1
  PS-Simulink Converter8/1 -> Mux3/1
  PS-Simulink Converter9/1 -> Mux3/2
  Mux3/1 -> [RphiANDdphiHip]
  Mux15/1 -> L GLU Golgi Tendon Organs3/1
  [RHipMomentR] -> L GLU Golgi Tendon Organs1/1
  L GLU Golgi Tendon Organs3/1 -> [RthetaANDdthetaHipR]
  L GLU Golgi Tendon Organs1/1 -> Simulink-PS Converter5/1
  Left Thigh/1 -> [LLLoad]
  Right Thigh/1 -> [RLLoad]
  [RAnklePos] -> "Left lateral d, v in body frame"/2
  [HATPosVel] -> "Right lateral d, v in body frame"/3, "Left lateral d, v in body frame"/3
  [psiHAT] -> "Left lateral d, v in body frame"/1, "Right lateral d, v in body frame"/1
  [LAnklePos] -> "Right lateral d, v in body frame"/2
  [RAnklePos] -> "Left sagittal d, v in body frame"/2
  [HATPosVel] -> "Left sagittal d, v in body frame"/3, "Right sagittal d, v in body frame"/3
  [psiHAT] -> "Right sagittal d, v in body frame"/1, "Left sagittal d, v in body frame"/1
  [LAnklePos] -> "Right sagittal d, v in body frame"/2
  "Left sagittal d, v in body frame"/1 -> [front_dv_L]
  "Right sagittal d, v in body frame"/1 -> [front_dv_R]
  "Left lateral d, v in body frame"/1 -> [side_dv_L]
  "Right lateral d, v in body frame"/1 -> L GLU Golgi Tendon Organs5/1
  Position Sensor14/1 -> [LKneePos]
  PS-Simulink Converter10/1 -> Mux15/1
  PS-Simulink Converter11/1 -> Mux15/2
  [LAnkleMoment] -> Simulink-PS Converter/1
  body pitch/roll/yaw in body frame --- x-axis: forward y-axis: leftward z-axis: parallel to gravity/3 -> [psiHAT]
  Position Sensor12/1 -> [LShankPos]
  Position Sensor10/1 -> [RShankPos]
  Position Velocity Sensor1/1 -> [LHipPosVel]
  Position Velocity Sensor2/1 -> [RHipPosVel]
  Position Velocity Sensor/1 -> [HATPosVel]
  [HATPosVel] -> body pitch/roll/yaw in body frame --- x-axis: forward y-axis: leftward z-axis: parallel to gravity/2
  [RHipPosVel] -> body pitch/roll/yaw in body frame --- x-axis: forward y-axis: leftward z-axis: parallel to gravity/3
  [LHipPosVel] -> body pitch/roll/yaw in body frame --- x-axis: forward y-axis: leftward z-axis: parallel to gravity/1
  body pitch/roll/yaw in body frame --- x-axis: forward y-axis: leftward z-axis: parallel to gravity/1 -> [phiANDdphiHAT]
  body pitch/roll/yaw in body frame --- x-axis: forward y-axis: leftward z-axis: parallel to gravity/2 -> [thetaANDdthetaHAT]
  [RHipMoment] -> Simulink-PS Converter4/1
  [LKneeMoment] -> Simulink-PS Converter1/1
  [RKneeMoment] -> Simulink-PS Converter6/1
  Right Foot/3 -> [RToePos]
  Right Foot/1 -> [RStance]
  Right Foot/2 -> [RGRF]
  Right Foot/4 -> [RHeelPos]
  Left Foot/4 -> [LHeelPos]
  Left Foot/2 -> [LGRF]
  Left Foot/1 -> [LStance]
  Left Foot/3 -> [LToePos]
  L GLU Golgi Tendon Organs5/1 -> [side_dv_R]
  [psiHAT] -> Right Foot/1
  [psiHAT] -> Left Foot/1
  Position Velocity Sensor3/1 -> [HATtopPosVel]
  connections:
  Solver Configuration/RConn1 -- Rigid Transform/LConn1 -- World Frame X-forward Y-lateral Z-up1/RConn1 -- TO: X-forward Y-up Z-lateral/RConn1 -- Mechanism Configuration/RConn1
  Rigid Transform/RConn1 -- Ground1/RConn1
  Bushing Joint/LConn1 -- TO: X-forward Y-up Z-lateral/LConn1
  Left Ankle joint/LConn2 -- Simulink-PS Converter/RConn1
  Left Ankle joint/RConn2 -- PS-Simulink Converter/LConn1
  Left Ankle joint/RConn3 -- PS-Simulink Converter1/LConn1
  Left Shank/RConn2 -- Position Sensor13/LConn1 -- Left Ankle joint/RConn1
  Position Sensor14/LConn1 -- Left Knee Joint/RConn1 -- Left Thigh/LConn1
  Simulink-PS Converter1/RConn1 -- Left Knee Joint/LConn2
  PS-Simulink Converter2/LConn1 -- Left Knee Joint/RConn2
  Left Knee Joint/RConn3 -- PS-Simulink Converter3/LConn1
  PS-Simulink Converter4/LConn1 -- Left Hip Joint/RConn2
  PS-Simulink Converter5/LConn1 -- Left Hip Joint/RConn3
  PS-Simulink Converter6/LConn1 -- Left Hip Joint/RConn4
  Simulink-PS Converter2/RConn1 -- Left Hip Joint/LConn2
  Simulink-PS Converter3/RConn1 -- Left Hip Joint/LConn3
  PS-Simulink Converter8/LConn1 -- Right Hip joint/RConn2
  Right Hip joint/RConn3 -- PS-Simulink Converter9/LConn1
  Right Hip joint/RConn4 -- PS-Simulink Converter10/LConn1
  Right Hip joint/RConn5 -- PS-Simulink Converter11/LConn1
  Simulink-PS Converter4/RConn1 -- Right Hip joint/LConn2
  Simulink-PS Converter5/RConn1 -- Right Hip joint/LConn3
  PS-Simulink Converter12/LConn1 -- Right Knee joint/RConn2
  PS-Simulink Converter13/LConn1 -- Right Knee joint/RConn3
  Position Sensor15/LConn1 -- Right Thigh/LConn1 -- Right Knee joint/RConn1
  Right Knee joint/LConn1 -- Right Shank/LConn1
  Position Sensor11/LConn1 -- Right Shank/RConn2 -- Right Ankle Joint/RConn1
  PS-Simulink Converter14/LConn1 -- Right Ankle Joint/RConn2
  PS-Simulink Converter15/LConn1 -- Right Ankle Joint/RConn3
  Simulink-PS Converter7/RConn1 -- Right Ankle Joint/LConn2
  Right Foot/LConn1 -- Right Ankle Joint/LConn1
  Right Hip joint/LConn1 -- Right Thigh/RConn1
  Left Shank/LConn1 -- Left Knee Joint/LConn1
  Left Hip Joint/LConn1 -- Left Thigh/RConn1
  HATs/LConn1 -- Rigid Transform5/LConn1 -- Rigid Transform4/LConn1 -- Left Hip Joint/RConn1 -- Position Velocity Sensor1/LConn1
  HATs/LConn2 -- Right Hip joint/RConn1 -- Position Velocity Sensor2/LConn1
  Simulink-PS Converter6/RConn1 -- Right Knee joint/LConn2
  Left Hip Joint/RConn5 -- PS-Simulink Converter7/LConn1
  HATs/RConn1 -- Position Velocity Sensor/LConn1
  Position Sensor10/LConn1 -- Right Shank/RConn1
  Position Sensor12/LConn1 -- Left Shank/RConn1
  Left Ankle joint/LConn1 -- Left Foot/LConn1
  Bushing Joint/RConn1 -- Left Foot/RConn1
  Whole Body side Tracking Camera/RConn1 -- Rigid Transform4/RConn1
  Whole Body front Tracking Camera/RConn1 -- Rigid Transform5/RConn1
  Position Velocity Sensor3/LConn1 -- HATs/RConn2

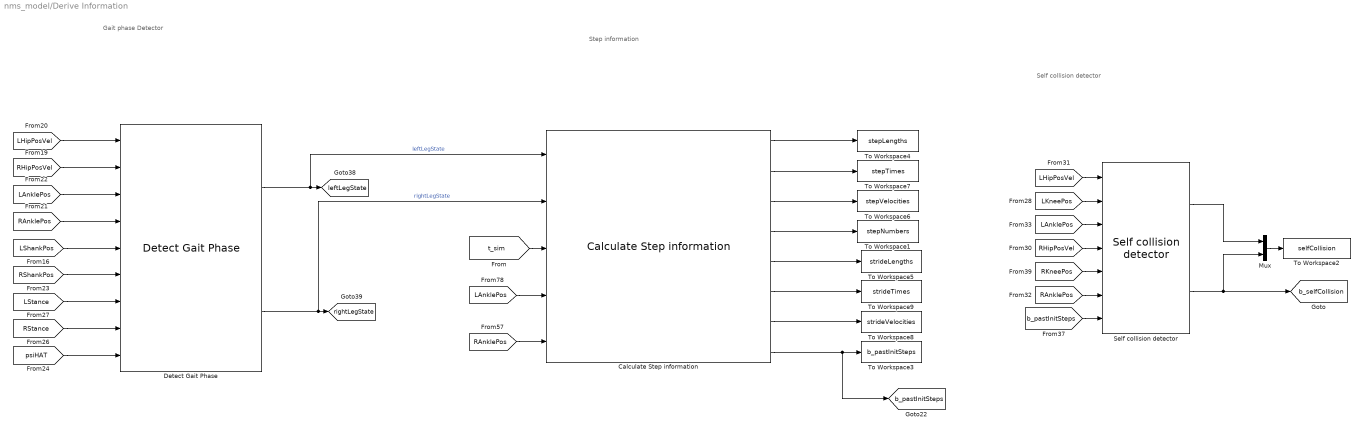
== system nms_model/Derive Information ==
  note: Self collision detector
  note: Gait phase Detector
  note: Step information
  Calculate Step information : NeuroMuscularLibrary/Calculate Step information  initiationSteps=innerOptSettings.initiationSteps
  Detect Gait Phase : NeuroMuscularLibrary/Detect Gait Phase  SystemSampleTime=-1  Latency=0  AutoFrameSizeCalculation=off
  Mux : Mux  Inputs=2
  Self collision detector : NeuroMuscularLibrary/Self collision detector  maxDist=innerOptSettings.minLimbDistance
  To Workspace1 : ToWorkspace  VariableName=stepNumbers  SaveFormat=Structure With Time  SampleTime=-1
  To Workspace2 : ToWorkspace  VariableName=selfCollision  SaveFormat=Structure With Time  SampleTime=dt_visual
  To Workspace3 : ToWorkspace  VariableName=b_pastInitSteps  SaveFormat=Structure With Time  SampleTime=-1
  To Workspace4 : ToWorkspace  VariableName=stepLengths  SaveFormat=Structure With Time  SampleTime=-1
  To Workspace5 : ToWorkspace  VariableName=strideLengths  SaveFormat=Structure With Time  SampleTime=-1
  To Workspace6 : ToWorkspace  VariableName=stepVelocities  SaveFormat=Structure With Time  SampleTime=-1
  To Workspace7 : ToWorkspace  VariableName=stepTimes  SaveFormat=Structure With Time  SampleTime=-1
  To Workspace8 : ToWorkspace  VariableName=strideVelocities  SaveFormat=Structure With Time  SampleTime=-1
  To Workspace9 : ToWorkspace  VariableName=strideTimes  SaveFormat=Structure With Time  SampleTime=-1
  tag scope: b_pastInitSteps=global, b_selfCollision=global, leftLegState=global, rightLegState=global
  wires:
  [RHipPosVel] -> Detect Gait Phase/2
  [LKneePos] -> Self collision detector/2
  [RHipPosVel] -> Self collision detector/4
  Mux/1 -> To Workspace2/1
  Self collision detector/2 -> [b_selfCollision], Mux/2
  [RAnklePos] -> Self collision detector/6
  Detect Gait Phase/1 -> Calculate Step information/1, [leftLegState]  "leftLegState"
  [LHipPosVel] -> Detect Gait Phase/1
  Self collision detector/1 -> Mux/1
  Detect Gait Phase/2 -> Calculate Step information/2, [rightLegState]  "rightLegState"
  [LHipPosVel] -> Self collision detector/1
  [b_pastInitSteps] -> Self collision detector/7
  [RStance] -> Detect Gait Phase/8
  [LStance] -> Detect Gait Phase/7
  [RShankPos] -> Detect Gait Phase/6
  [RAnklePos] -> Detect Gait Phase/4
  [psiHAT] -> Detect Gait Phase/9
  [RKneePos] -> Self collision detector/5
  [LAnklePos] -> Self collision detector/3
  [LShankPos] -> Detect Gait Phase/5
  [LAnklePos] -> Detect Gait Phase/3
  [RAnklePos] -> Calculate Step information/5
  Calculate Step information/1 -> To Workspace4/1
  Calculate Step information/3 -> To Workspace6/1
  [LAnklePos] -> Calculate Step information/4
  Calculate Step information/8 -> [b_pastInitSteps], To Workspace3/1
  Calculate Step information/4 -> To Workspace1/1
  [t_sim] -> Calculate Step information/3
  Calculate Step information/2 -> To Workspace7/1
  Calculate Step information/5 -> To Workspace5/1
  Calculate Step information/6 -> To Workspace9/1
  Calculate Step information/7 -> To Workspace8/1

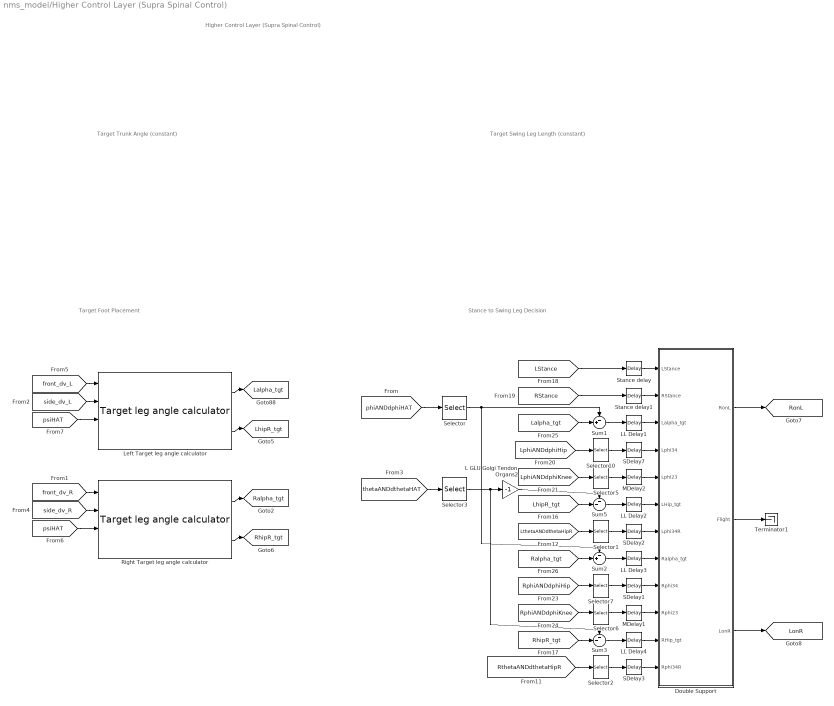
== system nms_model/Higher Control Layer (Supra Spinal Control) ==
  note: Target Foot Placement
  note: Target Swing Leg Length
      | (constant)
  note: Stance to Swing Leg Decision
  note: Target Trunk Angle
      | (constant)
  note: Higher Control Layer
      | (Supra Spinal Control)
  Double Support : Subsystem
  L GLU Golgi Tendon Organs2 : Gain  Gain=-1
  LL Delay1 : TransportDelay  DelayTime=LongLoopDelay/2  InitialOutput=initialTargetAngle
  LL Delay2 : TransportDelay  DelayTime=LongLoopDelay/2
  LL Delay3 : TransportDelay  DelayTime=LongLoopDelay/2  InitialOutput=initialTargetAngle
  LL Delay4 : TransportDelay  DelayTime=LongLoopDelay/2
  Left Target leg angle calculator : NeuroMuscularLibrary/Target leg angle calculator  simbiconLegAngle0=simbiconLegAngle0  simbiconGainD=simbiconGainD  simbiconGainV=simbiconGainV  simbiconLegAngle0_C=simbiconLegAngle0_C  simbiconGainD_C=simbiconGainD_C  simbiconGainV_C=simbiconGainV_C  headingGain=0  headingIntGain=0
  MDelay1 : TransportDelay  DelayTime=MidDelay
  MDelay2 : TransportDelay  DelayTime=MidDelay
  Right Target leg angle calculator : NeuroMuscularLibrary/Target leg angle calculator  simbiconLegAngle0=simbiconLegAngle0  simbiconGainD=simbiconGainD  simbiconGainV=simbiconGainV  simbiconLegAngle0_C=simbiconLegAngle0_C  simbiconGainD_C=simbiconGainD_C  simbiconGainV_C=simbiconGainV_C  headingGain=0  headingIntGain=0
  SDelay{1..3,7} (4 alike) : TransportDelay  DelayTime=ShortDelay
  Selector : Selector  InputPortWidth=2  IndexOptions=Index vector (dialog)  Indices=[1]  OutputSizes=1
  Selector{1..2,5..7,10} (6 alike) : Selector  InputPortWidth=2  IndexOptions=Index vector (dialog)  Indices=1  OutputSizes=1
  Selector3 : Selector  InputPortWidth=2  IndexOptions=Index vector (dialog)  Indices=[1]  OutputSizes=1
  Stance delay : TransportDelay  DelayTime=MidDelay
  Stance delay1 : TransportDelay  DelayTime=MidDelay
  Sum1 : Sum  Inputs=-+|
  Sum2 : Sum  Inputs=-+|
  Sum3 : Sum  Inputs=--|
  Sum5 : Sum  Inputs=--|
  Terminator1 : Terminator
  tag scope: Lalpha_tgt=global, LhipR_tgt=global, LonR=global, Ralpha_tgt=global, RhipR_tgt=global, RonL=global
  wires:
  [LphiANDdphiHip] -> Selector10/1
  [LphiANDdphiKnee] -> Selector5/1
  Selector10/1 -> SDelay7/1
  Selector5/1 -> MDelay2/1
  [RphiANDdphiHip] -> Selector7/1
  [RphiANDdphiKnee] -> Selector6/1
  Selector7/1 -> SDelay1/1
  Selector6/1 -> MDelay1/1
  Double Support/3(LonR) -> [LonR]
  Stance delay/1 -> Double Support/1(LStance)
  Stance delay1/1 -> Double Support/2(RStance)
  Double Support/1(RonL) -> [RonL]
  [LStance] -> Stance delay/1
  [RStance] -> Stance delay1/1
  Double Support/2(Flight) -> Terminator1/1
  LL Delay1/1 -> Double Support/3(Lalpha_tgt)
  LL Delay3/1 -> Double Support/8(Ralpha_tgt)
  SDelay7/1 -> Double Support/4(Lphi34)
  SDelay1/1 -> Double Support/9(Rphi34)
  MDelay2/1 -> Double Support/5(Lphi23)
  MDelay1/1 -> Double Support/10(Rphi23)
  Sum1/1 -> LL Delay1/1
  [Lalpha_tgt] -> Sum1/2
  Selector/1 -> Sum2/1, Sum1/1
  [Ralpha_tgt] -> Sum2/2
  Sum2/1 -> LL Delay3/1
  [LthetaANDdthetaHipR] -> Selector1/1
  Selector1/1 -> SDelay2/1
  SDelay2/1 -> Double Support/7(Lphi34R)
  LL Delay2/1 -> Double Support/6(LHip_tgt)
  Sum5/1 -> LL Delay2/1
  [LhipR_tgt] -> Sum5/2
  Selector3/1 -> L GLU Golgi Tendon Organs2/1, Sum3/1
  L GLU Golgi Tendon Organs2/1 -> Sum5/1
  [RthetaANDdthetaHipR] -> Selector2/1
  Selector2/1 -> SDelay3/1
  SDelay3/1 -> Double Support/12(Rphi34R)
  LL Delay4/1 -> Double Support/11(RHip_tgt)
  Sum3/1 -> LL Delay4/1
  [RhipR_tgt] -> Sum3/2
  [phiANDdphiHAT] -> Selector/1
  [thetaANDdthetaHAT] -> Selector3/1
  Right Target leg angle calculator/2 -> [RhipR_tgt]
  Right Target leg angle calculator/1 -> [Ralpha_tgt]
  Left Target leg angle calculator/2 -> [LhipR_tgt]
  Left Target leg angle calculator/1 -> [Lalpha_tgt]
  [side_dv_R] -> Right Target leg angle calculator/2
  [side_dv_L] -> Left Target leg angle calculator/2
  [front_dv_R] -> Right Target leg angle calculator/1
  [front_dv_L] -> Left Target leg angle calculator/1
  [psiHAT] -> Right Target leg angle calculator/3
  [psiHAT] -> Left Target leg angle calculator/3
